simulink model "ControleFF_trajetoria_D_integrado_RRR"  (R2020a)
settings: Solver=ode23  StartTime=0  StopTime=5  FixedStep=rate  RelTol=1e-3
values from neighbouring files (symbols this model uses):
  Beff = 50    [Ex4.m]    (also in initializeRobotParameters.m; plot_angular_positions.m; plot_angular_positions_RRR.m; testes.m)
  Jeff = 2.2    [Ex4.m]    (also in initializeRobotParameters.m = 0.5; plot_angular_positions.m = 0.5; plot_angular_positions_RRR.m = 0.5; testes.m = 0.5)
  K = 17.7    [Ex4.m]    (also in initializeRobotParameters.m = 0.785398163397; plot_angular_positions.m = 0.785398163397; plot_angular_positions_RRR.m = 0.785398163397; testes.m = 0.785398163397)
  Kd = (2*qsi*wn*Jeff - Beff)/K    (= -0.338983050847)    [Ex4.m]    (also in initializeRobotParameters.m = -44.5633840657; plot_angular_positions.m = -44.5633840657; plot_angular_positions_RRR.m = -44.5633840657; testes.m = -44.5633840657)
  Kp = (wn^2*Jeff)/K    (= 12.4293785311)    [Ex4.m]    (also in initializeRobotParameters.m = 143.239448783; plot_angular_positions.m = 143.239448783; plot_angular_positions_RRR.m = 143.239448783; testes.m = 143.239448783)
  N = 10    [Ex4.m]    (also in initializeRobotParameters.m = 3; plot_angular_positions.m = 3; plot_angular_positions_RRR.m = 3; testes.m = 3)
  r = 0.01    [Ex4.m]    (also in initializeRobotParameters.m = 1./[231.22*4 139.138 139.138 231.22 231.22]; plot_angular_positions.m = 1./[231.22*4 139.138 139.138 231.22 231.22]; plot_angular_positions_RRR.m = 1./[231.22*4 139.138 139.138]; testes.m = 1./[231.22*4 139.138 139.138 231.22 231.22])
  SP_theta = [0, 0, 0]    [Ex4.m]    (also in SP_theta.mat = [1.57079632679 0.0274016692563 0 0 0]; testeIntegracao.m = [0 0 0 0 0]; testes.m = [0,0,0,0,0])
libraries: simulink_extras x6
settings Model: Creator=Karoline  LastModifiedBy=lunet
settings DataIOCC: ReturnWorkspaceOutputs=off
settings DebuggingCC: ArithmeticOperatorsInVariantConditions=warning
settings SFSimCC: SimUseLocalCustomCode=off  CustomCodeUndefinedFunction=UseInterfaceOnly
settings RTWCC: RTWUseLocalCustomCode=off
settings CodeAppCC: StateflowObjectComments=on

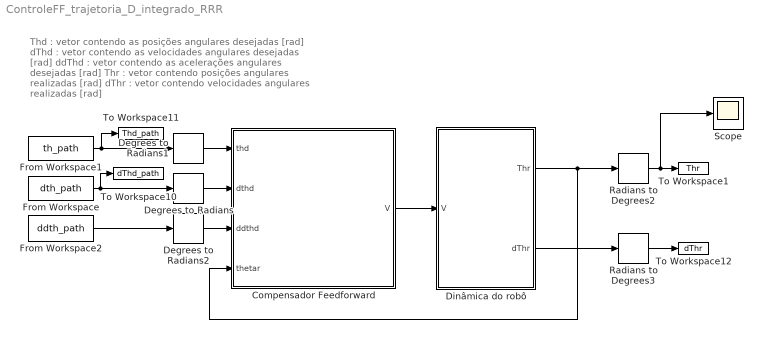
== system ControleFF_trajetoria_D_integrado_RRR ==
  note: Thd : vetor contendo as posições angulares desejadas [rad]
      | dThd : vetor contendo as velocidades angulares desejadas [rad]
      | ddThd : vetor contendo as acelerações angulares desejadas [rad]
      |
      | Thr : vetor contendo posições angulares realizadas [rad]
      | dThr : vetor contendo velocidades angulares realizadas [rad]
  Compensador Feedforward : Subsystem
  Degrees to Radians : simulink_extras/Transformations/Degrees to Radians
  Degrees to Radians1 : simulink_extras/Transformations/Degrees to Radians
  Degrees to Radians2 : simulink_extras/Transformations/Degrees to Radians
  Dinâmica do robô : Subsystem
  From Workspace : FromWorkspace  VariableName=dth_path
  From Workspace1 : FromWorkspace  VariableName=th_path
  From Workspace2 : FromWorkspace  VariableName=ddth_path
  Radians to Degrees2 : simulink_extras/Transformations/Radians to Degrees
  Radians to Degrees3 : simulink_extras/Transformations/Radians to Degrees
  Scope : Scope
  To Workspace1 : ToWorkspace  VariableName=Thr  SaveFormat=Structure With Time  SampleTime=-1
  To Workspace10 : ToWorkspace  VariableName=dThd_path  SaveFormat=Structure With Time  SampleTime=-1
  To Workspace11 : ToWorkspace  VariableName=Thd_path  SaveFormat=Structure With Time  SampleTime=-1
  To Workspace12 : ToWorkspace  VariableName=dThr  SaveFormat=Structure With Time  SampleTime=-1
  wires:
  Dinâmica do robô/2("dThr ") -> Radians to Degrees3/1
  Compensador Feedforward/1(V) -> Dinâmica do robô/1(V)
  Dinâmica do robô/1(Thr) -> Compensador Feedforward/4(thetar), Radians to Degrees2/1
  From Workspace2/1 -> Degrees to Radians2/1
  Degrees to Radians2/1 -> Compensador Feedforward/3(ddthd)
  From Workspace/1 -> Degrees to Radians/1, To Workspace10/1
  From Workspace1/1 -> Degrees to Radians1/1, To Workspace11/1
  Degrees to Radians1/1 -> Compensador Feedforward/1(thd)
  Degrees to Radians/1 -> Compensador Feedforward/2(dthd)
  Radians to Degrees3/1 -> To Workspace12/1
  Radians to Degrees2/1 -> Scope/1, To Workspace1/1

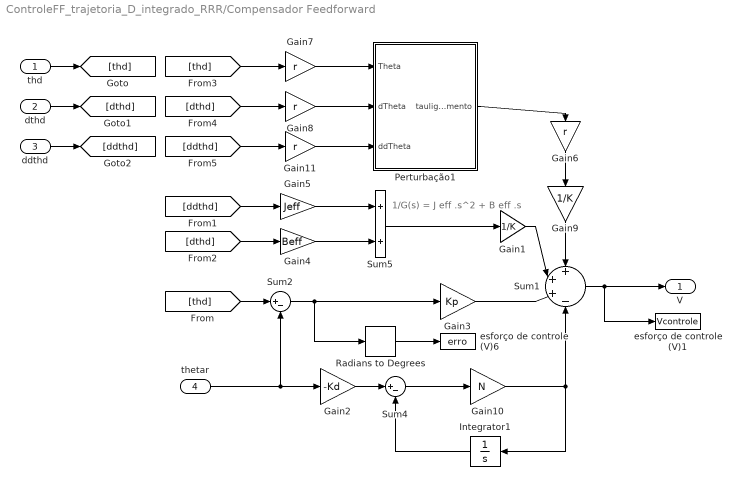
== system ControleFF_trajetoria_D_integrado_RRR/Compensador Feedforward ==
  note: 1/G(s) = J eff .s^2 + B eff .s
  thd : Inport
  dthd : Inport  Port=2
  ddthd : Inport  Port=3
  thetar : Inport  Port=4
  Gain1 : Gain  Gain=1/K
  Gain10 : Gain  Gain=N
  Gain{6..8,11} (4 alike) : Gain  Gain=r
  Gain2 : Gain  Gain=-Kd
  Gain3 : Gain  Gain=Kp
  Gain4 : Gain  Gain=Beff
  Gain5 : Gain  Gain=Jeff
  Gain9 : Gain  Gain=1/K
  Integrator1 : Integrator
  Perturbação1 : Subsystem
  Radians to Degrees : simulink_extras/Transformations/Radians to Degrees
  Sum1 : Sum  Inputs=+|+|+|-
  Sum2 : Sum  Inputs=|+-
  Sum4 : Sum  Inputs=|+-
  Sum5 : Sum
  esforço de controle (V)1 : ToWorkspace  VariableName=Vcontrole  SaveFormat=Structure With Time  SampleTime=-1
  esforço de controle (V)6 : ToWorkspace  VariableName=erro  SaveFormat=Structure With Time  SampleTime=-1
  V : Outport  VectorParamsAs1DForOutWhenUnconnected=off
  wires:
  Gain2/1 -> Sum4/1
  thetar/1 -> Sum2/2, Gain2/1
  Sum4/1 -> Gain10/1
  Integrator1/1 -> Sum4/2
  Gain10/1 -> Sum1/4, Integrator1/1
  Gain4/1 -> Sum5/2
  Gain5/1 -> Sum5/1
  Sum5/1 -> Gain1/1
  Gain8/1 -> Perturbação1/2(dTheta)
  Gain7/1 -> Perturbação1/1(Theta)
  [thd] -> Gain7/1
  [dthd] -> Gain8/1
  Perturbação1/1(tauligamento) -> Gain6/1
  Gain6/1 -> Gain9/1
  Gain9/1 -> Sum1/1
  thd/1 -> [thd]
  [thd] -> Sum2/1
  ddthd/1 -> [ddthd]
  [ddthd] -> Gain5/1
  dthd/1 -> [dthd]
  [dthd] -> Gain4/1
  Gain3/1 -> Sum1/3
  Gain1/1 -> Sum1/2
  Sum1/1 -> esforço de controle (V)1/1, V/1
  Radians to Degrees/1 -> esforço de controle (V)6/1
  Sum2/1 -> Radians to Degrees/1, Gain3/1
  [ddthd] -> Gain11/1
  Gain11/1 -> Perturbação1/3(ddTheta)

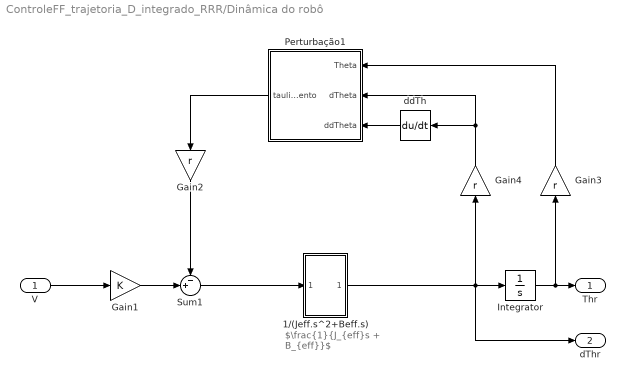
== system ControleFF_trajetoria_D_integrado_RRR/Dinâmica do robô ==
  note: $\frac{1}{J_{eff}s + B_{eff}}$
  V : Inport
  1/(Jeff.s^2+Beff.s) : Subsystem
  Gain1 : Gain  Gain=K
  Gain2 : Gain  Gain=r
  Gain3 : Gain  Gain=r
  Gain4 : Gain  Gain=r
  Integrator : Integrator  InitialCondition=SP_theta*pi/180
  Perturbação1 : Subsystem
  Sum1 : Sum  Inputs=-+|
  ddTh : Derivative
  Thr : Outport  VectorParamsAs1DForOutWhenUnconnected=off
  "dThr " : Outport  Port=2  VectorParamsAs1DForOutWhenUnconnected=off
  wires:
  Perturbação1/1(tauligamento) -> Gain2/1
  Gain1/1 -> Sum1/2
  Integrator/1 -> Thr/1, Gain3/1
  V/1 -> Gain1/1
  Gain2/1 -> Sum1/1
  ddTh/1 -> Perturbação1/3(ddTheta)
  Gain3/1 -> Perturbação1/1(Theta)
  Gain4/1 -> Perturbação1/2(dTheta), ddTh/1
  1/(Jeff.s^2+Beff.s)/1(Out1) -> Integrator/1, "dThr "/1, Gain4/1
  Sum1/1 -> 1/(Jeff.s^2+Beff.s)/1(In1)

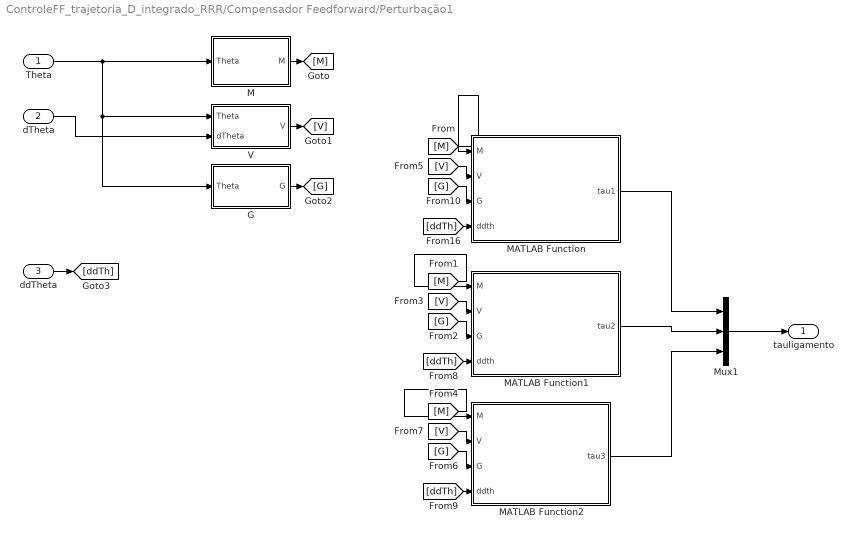
== system ControleFF_trajetoria_D_integrado_RRR/Compensador Feedforward/Perturbação1 ==
  Theta : Inport
  dTheta : Inport  Port=2
  ddTheta : Inport  Port=3
  G : Subsystem
  M : Subsystem
  MATLAB Function : MATLAB Function  TreatAsAtomicUnit=on
  MATLAB Function1 : MATLAB Function  TreatAsAtomicUnit=on
  MATLAB Function2 : MATLAB Function  TreatAsAtomicUnit=on
  Mux1 : Mux  Inputs=3
  V : Subsystem
  tauligamento : Outport  VectorParamsAs1DForOutWhenUnconnected=off
  wires:
  dTheta/1 -> V/2(dTheta)
  Theta/1 -> M/1(Theta), V/1(Theta), G/1(Theta)
  ddTheta/1 -> [ddTh]
  M/1(M) -> [M]
  V/1(V) -> [V]
  G/1(G) -> [G]
  [V] -> MATLAB Function/2(V)
  [M] -> MATLAB Function/1(M)
  [G] -> MATLAB Function/3(G)
  [V] -> MATLAB Function1/2(V)
  [M] -> MATLAB Function1/1(M)
  [G] -> MATLAB Function1/3(G)
  [M] -> MATLAB Function2/1(M)
  [V] -> MATLAB Function2/2(V)
  [G] -> MATLAB Function2/3(G)
  [ddTh] -> MATLAB Function/4(ddth)
  [ddTh] -> MATLAB Function1/4(ddth)
  [ddTh] -> MATLAB Function2/4(ddth)
  Mux1/1 -> tauligamento/1
  MATLAB Function/1(tau1) -> Mux1/1
  MATLAB Function1/1(tau2) -> Mux1/2
  MATLAB Function2/1(tau3) -> Mux1/3

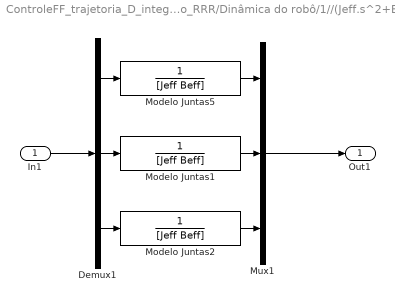
== system ControleFF_trajetoria_D_integrado_RRR/Dinâmica do robô/1//(Jeff.s^2+Beff.s) ==
  In1 : Inport
  Demux1 : Demux  Outputs=3
  Modelo Juntas1 : TransferFcn  Denominator=[Jeff Beff]
  Modelo Juntas2 : TransferFcn  Denominator=[Jeff Beff]
  Modelo Juntas5 : TransferFcn  Denominator=[Jeff Beff]
  Mux1 : Mux  Inputs=3
  Out1 : Outport
  wires:
  Modelo Juntas5/1 -> Mux1/1
  Demux1/1 -> Modelo Juntas5/1
  Modelo Juntas2/1 -> Mux1/3
  Demux1/3 -> Modelo Juntas2/1
  Modelo Juntas1/1 -> Mux1/2
  Demux1/2 -> Modelo Juntas1/1
  Mux1/1 -> Out1/1
  In1/1 -> Demux1/1

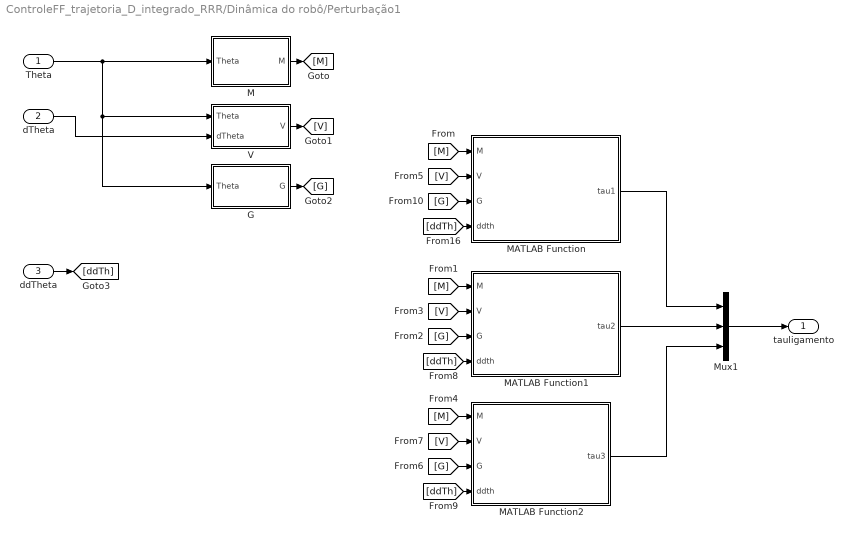
== system ControleFF_trajetoria_D_integrado_RRR/Dinâmica do robô/Perturbação1 ==
  Theta : Inport
  dTheta : Inport  Port=2
  ddTheta : Inport  Port=3
  G : Subsystem
  M : Subsystem
  MATLAB Function : MATLAB Function  TreatAsAtomicUnit=on
  MATLAB Function1 : MATLAB Function  TreatAsAtomicUnit=on
  MATLAB Function2 : MATLAB Function  TreatAsAtomicUnit=on
  Mux1 : Mux  Inputs=3
  V : Subsystem
  tauligamento : Outport  VectorParamsAs1DForOutWhenUnconnected=off
  wires:
  dTheta/1 -> V/2(dTheta)
  Theta/1 -> M/1(Theta), V/1(Theta), G/1(Theta)
  ddTheta/1 -> [ddTh]
  M/1(M) -> [M]
  V/1(V) -> [V]
  G/1(G) -> [G]
  [V] -> MATLAB Function/2(V)
  [M] -> MATLAB Function/1(M)
  [G] -> MATLAB Function/3(G)
  [V] -> MATLAB Function1/2(V)
  [M] -> MATLAB Function1/1(M)
  [G] -> MATLAB Function1/3(G)
  [M] -> MATLAB Function2/1(M)
  [V] -> MATLAB Function2/2(V)
  [G] -> MATLAB Function2/3(G)
  [ddTh] -> MATLAB Function/4(ddth)
  [ddTh] -> MATLAB Function1/4(ddth)
  [ddTh] -> MATLAB Function2/4(ddth)
  Mux1/1 -> tauligamento/1
  MATLAB Function/1(tau1) -> Mux1/1
  MATLAB Function1/1(tau2) -> Mux1/2
  MATLAB Function2/1(tau3) -> Mux1/3

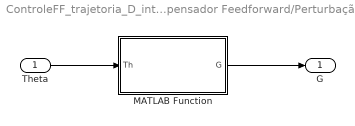
== system ControleFF_trajetoria_D_integrado_RRR/Compensador Feedforward/Perturbação1/G ==
  Theta : Inport
  MATLAB Function : MATLAB Function  TreatAsAtomicUnit=on
  G : Outport  VectorParamsAs1DForOutWhenUnconnected=off
  wires:
  Theta/1 -> MATLAB Function/1(Th)
  MATLAB Function/1(G) -> G/1

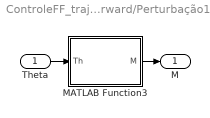
== system ControleFF_trajetoria_D_integrado_RRR/Compensador Feedforward/Perturbação1/M ==
  Theta : Inport
  MATLAB Function3 : MATLAB Function  TreatAsAtomicUnit=on
  M : Outport  VectorParamsAs1DForOutWhenUnconnected=off
  wires:
  Theta/1 -> MATLAB Function3/1(Th)
  MATLAB Function3/1(M) -> M/1

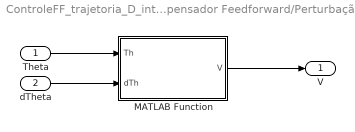
== system ControleFF_trajetoria_D_integrado_RRR/Compensador Feedforward/Perturbação1/V ==
  Theta : Inport
  dTheta : Inport  Port=2
  MATLAB Function : MATLAB Function  TreatAsAtomicUnit=on
  V : Outport  VectorParamsAs1DForOutWhenUnconnected=off
  wires:
  Theta/1 -> MATLAB Function/1(Th)
  MATLAB Function/1(V) -> V/1
  dTheta/1 -> MATLAB Function/2(dTh)

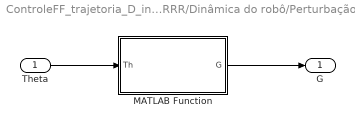
== system ControleFF_trajetoria_D_integrado_RRR/Dinâmica do robô/Perturbação1/G ==
  Theta : Inport
  MATLAB Function : MATLAB Function  TreatAsAtomicUnit=on
  G : Outport  VectorParamsAs1DForOutWhenUnconnected=off
  wires:
  Theta/1 -> MATLAB Function/1(Th)
  MATLAB Function/1(G) -> G/1

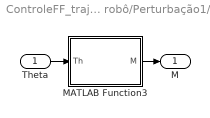
== system ControleFF_trajetoria_D_integrado_RRR/Dinâmica do robô/Perturbação1/M ==
  Theta : Inport
  MATLAB Function3 : MATLAB Function  TreatAsAtomicUnit=on
  M : Outport  VectorParamsAs1DForOutWhenUnconnected=off
  wires:
  Theta/1 -> MATLAB Function3/1(Th)
  MATLAB Function3/1(M) -> M/1

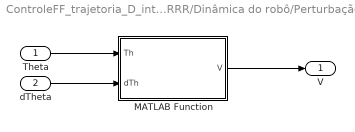
== system ControleFF_trajetoria_D_integrado_RRR/Dinâmica do robô/Perturbação1/V ==
  Theta : Inport
  dTheta : Inport  Port=2
  MATLAB Function : MATLAB Function  TreatAsAtomicUnit=on
  V : Outport  VectorParamsAs1DForOutWhenUnconnected=off
  wires:
  Theta/1 -> MATLAB Function/1(Th)
  MATLAB Function/1(V) -> V/1
  dTheta/1 -> MATLAB Function/2(dTh)

== matlab function ControleFF_trajetoria_D_integrado_RRR/Compensador Feedforward/Perturbação1/MATLAB Function2 ==
  data: M input; V input; tau3 output; G input; ddth input
function tau3  = calcul_dk3(M, V, G, ddth)



% tau3 = m31*ddth1 + m32*ddth2 + v3 + g3;
tau3 = M(3,1)*ddth(1) + M(3,2)*ddth(2) + V(3) + G(3);

== matlab function ControleFF_trajetoria_D_integrado_RRR/Compensador Feedforward/Perturbação1/V/MATLAB Function ==
  data: Th input; V output; dTh input
function V = calcul_V(Th,dTh)

th1 = Th(1);
th2 = Th(2);
th3 = Th(3);

dth1 = dTh(1);
dth2 = dTh(2);
dth3 = dTh(3);

V =[-(33*dth2^2*sin(th2))/40 - (33*dth1*dth2*sin(th2))/20;...
    (33*dth1^2*sin(th2))/40;...
    0];

== matlab function ControleFF_trajetoria_D_integrado_RRR/Dinâmica do robô/Perturbação1/V/MATLAB Function ==
  data: Th input; V output; dTh input
function V = calcul_V(Th,dTh)

th1 = Th(1);
th2 = Th(2);
th3 = Th(3);

dth1 = dTh(1);
dth2 = dTh(2);
dth3 = dTh(3);

V =[-(33*dth2^2*sin(th2))/40 - (33*dth1*dth2*sin(th2))/20;...
    (33*dth1^2*sin(th2))/40;...
    0];

== matlab function ControleFF_trajetoria_D_integrado_RRR/Dinâmica do robô/Perturbação1/G/MATLAB Function ==
  data: Th input; G output
function G = calcul_G(Th)

th1 = Th(1);
th2 = Th(2);
th3 = Th(3);

G = [(1617*cos(th1 + th2))/100 + (3871*cos(th1))/100;...
    (1617*cos(th1 + th2))/100;...
    0];

== matlab function ControleFF_trajetoria_D_integrado_RRR/Dinâmica do robô/Perturbação1/MATLAB Function1 ==
  data: M input; V input; tau2 output; G input; ddth input
function tau2  = calcul_dk2(M,V,G,ddth)


% tau2 = m21*ddth1 + m23*ddth3 + v2 + g2;
tau2 = M(2,1)*ddth(1) + M(2,3)*ddth(3) + V(2) + G(2);

== matlab function ControleFF_trajetoria_D_integrado_RRR/Dinâmica do robô/Perturbação1/MATLAB Function ==
  data: M input; V input; tau1 output; G input; ddth input
function tau1  = calcul_dk1(M,V,G,ddth)


% tau1 = m12*ddth2 + m13*ddth3 + v1 + g1;
tau1 = M(1,2)*ddth(2) + M(1,3)*ddth(3) + V(1) + G(1);

== matlab function ControleFF_trajetoria_D_integrado_RRR/Dinâmica do robô/Perturbação1/MATLAB Function2 ==
  data: M input; V input; tau3 output; G input; ddth input
function tau3  = calcul_dk3(M, V, G, ddth)



% tau3 = m31*ddth1 + m32*ddth2 + v3 + g3;
tau3 = M(3,1)*ddth(1) + M(3,2)*ddth(2) + V(3) + G(3);

== matlab function ControleFF_trajetoria_D_integrado_RRR/Dinâmica do robô/Perturbação1/M/MATLAB Function3 ==
  data: Th input; M output
function M = calcul_M(Th)

th1 = Th(1);
th2 = Th(2);
th3 = Th(3);

M = [(33*cos(th2))/20 + 29/10, (33*cos(th2))/40 + 37/40, 1/10;...
     (33*cos(th2))/40 + 37/40,                    37/40, 1/10;...
                         1/10,                     1/10, 1/10];

== matlab function ControleFF_trajetoria_D_integrado_RRR/Compensador Feedforward/Perturbação1/G/MATLAB Function ==
  data: Th input; G output
function G = calcul_G(Th)

th1 = Th(1);
th2 = Th(2);
th3 = Th(3);

G = [(1617*cos(th1 + th2))/100 + (3871*cos(th1))/100;...
    (1617*cos(th1 + th2))/100;...
    0];

== matlab function ControleFF_trajetoria_D_integrado_RRR/Compensador Feedforward/Perturbação1/M/MATLAB Function3 ==
  data: Th input; M output
function M = calcul_M(Th)

th1 = Th(1);
th2 = Th(2);
th3 = Th(3);

M = [(33*cos(th2))/20 + 29/10, (33*cos(th2))/40 + 37/40, 1/10;...
     (33*cos(th2))/40 + 37/40,                    37/40, 1/10;...
                         1/10,                     1/10, 1/10];

== matlab function ControleFF_trajetoria_D_integrado_RRR/Compensador Feedforward/Perturbação1/MATLAB Function ==
  data: M input; V input; tau1 output; G input; ddth input
function tau1  = calcul_dk1(M,V,G,ddth)


% tau1 = m12*ddth2 + m13*ddth3 + v1 + g1;
tau1 = M(1,2)*ddth(2) + M(1,3)*ddth(3) + V(1) + G(1);

== matlab function ControleFF_trajetoria_D_integrado_RRR/Compensador Feedforward/Perturbação1/MATLAB Function1 ==
  data: M input; V input; tau2 output; G input; ddth input
function tau2  = calcul_dk2(M,V,G,ddth)


% tau2 = m21*ddth1 + m23*ddth3 + v2 + g2;
tau2 = M(2,1)*ddth(1) + M(2,3)*ddth(3) + V(2) + G(2);
